simulink model "Hospital"  (R2020b)
settings: Solver=VariableStepAuto  StartTime=0.0  StopTime=10.0  RelTol=1e-3
libraries: dspstat3 x5
(part 2 of 2)

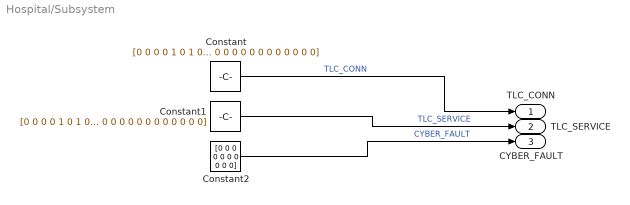
== system Hospital/Subsystem ==
  Constant : Constant  Value=[0 0 0 0 1 0 1 0 0 0 0 0 0 0 0 0 0 0 0 0]
  Constant1 : Constant  Value=[0 0 0 0 1 0 1 0 0 0 0 0 0 0 0 0 0 0 0 0]
  Constant2 : Constant  Value=[0 0 0 0 0 0 0 0 0 0]
  TLC_CONN : Outport
  TLC_SERVICE : Outport  Port=2
  CYBER_FAULT : Outport  Port=3
  wires:
  Constant2/1 -> CYBER_FAULT/1  "CYBER_FAULT"
  Constant/1 -> TLC_CONN/1  "TLC_CONN"
  Constant1/1 -> TLC_SERVICE/1  "TLC_SERVICE"
